simulink model "essai"  (R2016a)
settings: Solver=VariableStepAuto  StartTime=0.0  StopTime=10  RelTol=1e-3
values from neighbouring files (symbols this model uses):
  F1 = -acker(A,B,P1)    [Data.m]    (also in Q5.m)
  G = k*(s+c)/(s+a)/(s+b)/(s+b)    [Data.m]    (also in Q5.m)
  K1 = acker(A',C',Po1)'    [Data.m]    (also in Q5.m)
  K1_ = minreal(K1_,0.0001)    [Data.m]
  Reg1 = tf(ss(A+B*F1-K1*C, K1, -F1,0))    [Data.m]    (also in Q5.m = minreal(tf(ss(A+B*F1-K1*C, K1, -F1,0)),0.01))
undefined symbols (not defined in the file or in its folder): A, B, C
libraries: cstblocks x2
settings Model: Creator=NAD  LastModifiedBy=NAD

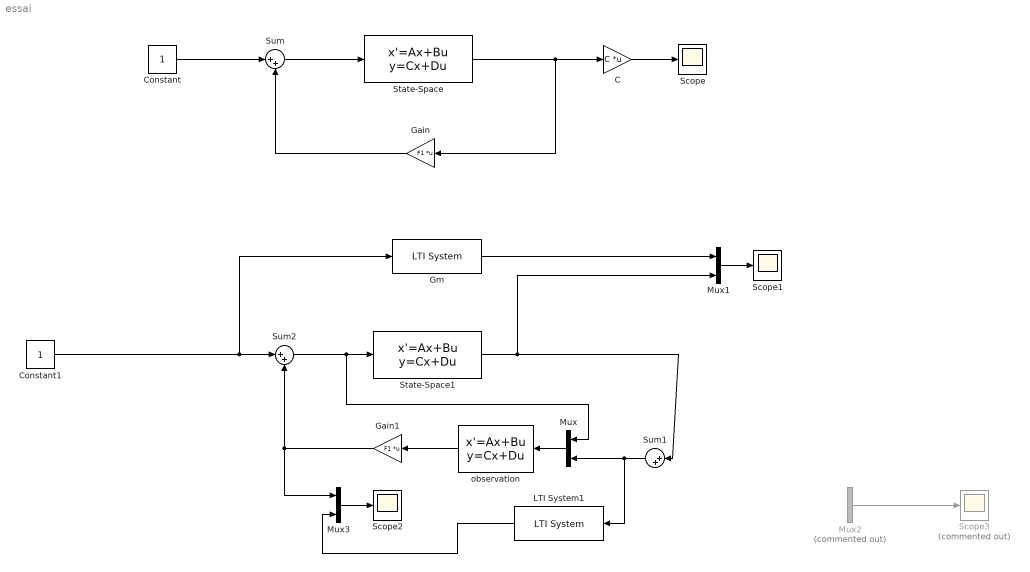
== system essai ==
  C : Gain  Gain=C  Multiplication=Matrix(K*u) (u vector)
  Constant : Constant
  Constant1 : Constant
  Gain : Gain  Gain=F1  Multiplication=Matrix(K*u) (u vector)
  Gain1 : Gain  Gain=F1  Multiplication=Matrix(K*u) (u vector)
  Gm : cstblocks/LTI System  sys=G*K1_/(1+G*Reg1)  IC=[]
  LTI System1 : cstblocks/LTI System  sys=-Reg1  IC=[]
  Mux : Mux  Inputs=2
  Mux1 : Mux  Inputs=2
  Mux2 : Mux  Commented=on  Inputs=2
  Mux3 : Mux  Inputs=2
  Scope : Scope
  Scope1 : Scope
  Scope2 : Scope
  Scope3 : Scope  Commented=on
  State-Space : StateSpace  A=A  B=B  C=eye(3,3)  D=[0;0;0]  X0=0
  State-Space1 : StateSpace  A=A  B=B  C=C  D=0  X0=0
  Sum : Sum  Inputs=|++
  Sum1 : Sum  Inputs=|++
  Sum2 : Sum  Inputs=|++
  observation : StateSpace  A=A-K1*C  B=[B , K1]  C=eye(3,3)  D=zeros(3,2)  X0=0
  wires:
  Sum/1 -> State-Space/1
  State-Space/1 -> C/1, Gain/1
  Gain/1 -> Sum/2
  Constant/1 -> Sum/1
  C/1 -> Scope/1
  Gain1/1 -> Sum2/2, Mux3/1
  Mux2/1 -> Scope3/1
  observation/1 -> Gain1/1
  Sum2/1 -> State-Space1/1, Mux/1
  Sum1/1 -> LTI System1/1, Mux/2
  State-Space1/1 -> Mux1/2, Sum1/1
  Mux/1 -> observation/1
  Gm/1 -> Mux1/1
  Mux1/1 -> Scope1/1
  Mux3/1 -> Scope2/1
  LTI System1/1 -> Mux3/2
  Constant1/1 -> Gm/1, Sum2/1
